simulink model "SSModel3D"  (R2016b)
settings: Solver=VariableStepAuto  StartTime=0.0  StopTime=3  RelTol=1e-3
values from neighbouring files (symbols this model uses):
  A3D = [ z3 F z3 ... (first row only)    [Cube3D.m]
  B3D = [ z3 ... (first row only)    [Cube3D.m]
  C3D = eye(9)    [Cube3D.m]
  D3D = zeros(9,3)    [Cube3D.m]
  K3D = [-5 -7 -5 -1 -1 -1 0 0 0]    [Cube3D.m]
settings Model: Creator=Will  LastModifiedBy=Will

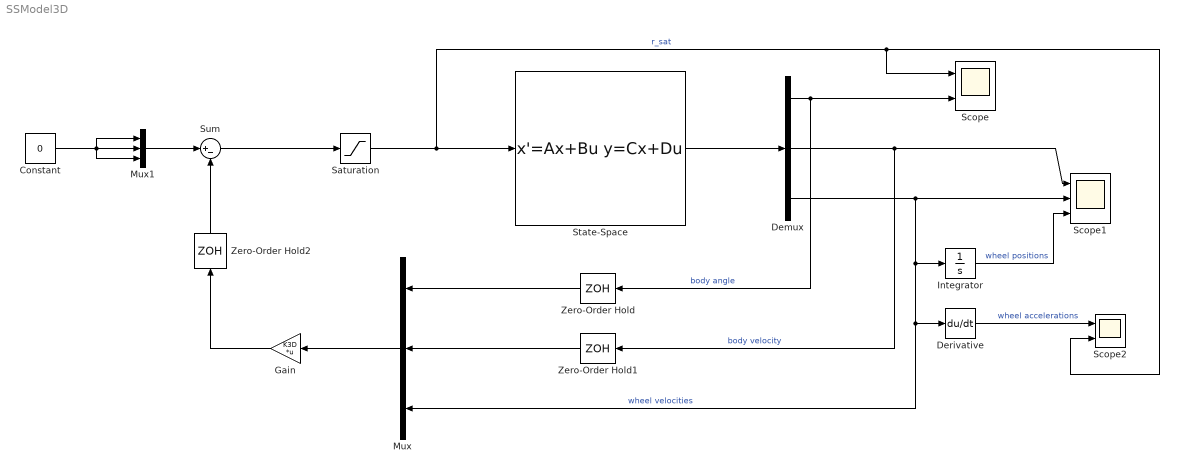
== system SSModel3D ==
  Constant : Constant  Value=0
  Demux : Demux  Outputs=3
  Derivative : Derivative
  Gain : Gain  Gain=K3D  Multiplication=Matrix(K*u)
  Integrator : Integrator
  Mux : Mux  Inputs=3
  Mux1 : Mux  Inputs=3
  Saturation : Saturate  UpperLimit=6  LowerLimit=-6
  Scope : Scope  NumInputPorts=2
  Scope1 : Scope  NumInputPorts=3
  Scope2 : Scope  NumInputPorts=2
  State-Space : StateSpace  A=A3D  B=B3D  C=C3D  D=D3D  X0=[.01 -.01 0 0 0 0 0 0 0]  ContinuousStateAttributes={'alpha', 'beta', 'gamma', 'alpha_dot', 'beta_dot', 'gamma_dot', 'omega1', 'omega2', 'omega3'}
  Sum : Sum  Inputs=|+-
  Zero-Order Hold : ZeroOrderHold  SampleTime=1/100
  Zero-Order Hold1 : ZeroOrderHold  SampleTime=1/100
  Zero-Order Hold2 : ZeroOrderHold  SampleTime=.005
  wires:
  State-Space/1 -> Demux/1
  Demux/1 -> Scope/2, Zero-Order Hold/1  "body angle"
  Demux/2 -> Zero-Order Hold1/1, Scope1/1  "body velocity"
  Demux/3 -> Integrator/1, Derivative/1, Mux/3, Scope1/2  "wheel velocities"
  Mux/1 -> Gain/1
  Sum/1 -> Saturation/1
  Gain/1 -> Zero-Order Hold2/1
  Constant/1 -> Mux1/1, Mux1/3, Mux1/2
  Mux1/1 -> Sum/1
  Saturation/1 -> Scope2/2, Scope/1, State-Space/1  "r_sat"
  Zero-Order Hold/1 -> Mux/1
  Zero-Order Hold1/1 -> Mux/2
  Zero-Order Hold2/1 -> Sum/2
  Integrator/1 -> Scope1/3  "wheel positions"
  Derivative/1 -> Scope2/1  "wheel accelerations"
